simulink model "SRF_DDSRF_Simulink_Imperix"  (R2025a)
settings: Solver=ode45  StartTime=0.0  StopTime=0.3  RelTol=1e-3
PreLoadFcn:
  | % --- DO NOT REMOVE THIS CODE (2024.2.b2) ---
  |     % create Simulink variants
  |     if not(exist('variant_simulation', 'var'))
  |         variant_simulation = Simulink.Variant('SIMULINK_MODE==0');
  |     end
  |     if not(exist('variant_generation', 'var'))
  |         variant_generation = Simulink.Variant('SIMULINK_MODE==1');
  |     end
  | 
  |     % check SDK version
  |     required_lib_version = 3900.3;
  |     required_lib_ver_str = '2024.2.beta2';
  |     lib_path = [getenv('IX_SIMULINK_ACG_BB_3') '\simulink\blocks\BoomBox.slx'];
  |     if exist(lib_path, 'file')
  |         lib_version = str2double(Simulink.MDLInfo(lib_path).ModelVersion); % fullpath to avoid getting shadowing files
  |         if lib_version < required_lib_version || isnan(lib_version)
  |             error(['The model ''' bdroot ''' has been saved with a more recent version of ACG SDK (' required_lib_ver_str ') and might not work as expected. <a href="matlab:private_end_string = ''--- PLACE YOUR CODE BELOW THIS LINE ---'';private_fcn = get_param(bdroot, ''PreLoadFcn'');private_end_index = strfind(private_fcn, private_end_string);set_param(bdroot, ''PreLoadFcn'', strtrim(private_fcn(private_end_index(end)+length(private_end_string):end)));private_fcn = get_param(bdroot, ''PostLoadFcn'');private_end_index = strfind(private_fcn, private_end_string);set_param(bdroot, ''PostLoadFcn'', strtrim(private_fcn(private_end_index(end)+length(private_end_string):end)));private_fcn = get_param(bdroot, ''InitFcn'');private_end_index = strfind(private_fcn, private_end_string);set_param(bdroot, ''InitFcn'', strtrim(private_fcn(private_end_index(end)+length(private_end_string):end)));clear private_end_string private_fcn private_end_index;open(bdroot);">Click here</a> to continue anyway, or download the latest version of the SDK at <a href="www.imperix.com/downloads">www.imperix.ch/downloads</a>.']);
  |         end
  |     elseif exist(getenv('IX_SIMULINK_ACG_BB_3'), 'dir')
  |         error(['Library file for imperix ACG SDK not found in path ''' lib_path '''. Please try to re-install ACG SDK (<a href="www.imperix.com/downloads">www.imperix.ch/downloads</a>).']);
  |     else
  |         error('ACG SDK is not installed on this computer and the model will not work as expected. Please download ACG SDK at <a href="www.imperix.com/downloads">www.imperix.ch/downloads</a>, install it, and reopen the model.');
  |     end
  |     clear required_lib_version required_lib_ver_str lib_path lib_version;
  | 
  |     ix_acg_path = getenv('IX_SIMULINK_ACG_BB_3');
  |     addpath(fullfile(ix_acg_path, 'simulink\target'));
  |     addpath(fullfile(ix_acg_path, 'simulink\blocks'));
  |     addpath(fullfile(ix_acg_path, 'simulink\functions'));
  |     sl_refresh_customizations;
  |     clear ix_acg_path;
  | 
  |     % The SIMULINK_MODE variable is created in the base
  |     % workspace in the PostLoadFcn from the block whose id is kb0101
  |     % All opened models share a common variant configuration.
  | 
  |     Model_PreLoadFcn(bdroot);
  | % --- PLACE YOUR CODE BELOW THIS LINE ---
PostLoadFcn:
  | % --- DO NOT REMOVE THIS CODE (2024.2.b2) ---
  |     % change the execution mode of simulink depending on the radio button:
  |     if(strcmp('Automated Code Generation',get_param(Find_imperix_blocks(bdroot,'Configuration'),'SLMODE')))
  |         assignin('base', 'SIMULINK_MODE', 1);
  |     else
  |         assignin('base', 'SIMULINK_MODE', 0);
  |     end
  | 
  |     Model_PostLoadFcn(bdroot);
  | % --- PLACE YOUR CODE BELOW THIS LINE ---
InitFcn:
  | % --- DO NOT REMOVE THIS CODE (2024.2.b2) ---
  |     % check SDK version
  |     required_lib_version = 3900.3;
  |     required_lib_ver_str = '2024.2.beta2';
  |     lib_path = [getenv('IX_SIMULINK_ACG_BB_3') '\simulink\blocks\BoomBox.slx'];
  |     if exist(lib_path, 'file')
  |         lib_version = str2double(Simulink.MDLInfo(lib_path).ModelVersion); % fullpath to avoid getting shadowing files
  |         if lib_version < required_lib_version || isnan(lib_version)
  |             error(['The model ''' bdroot ''' has been saved with a more recent version of ACG SDK (' required_lib_ver_str ') and might not work as expected. <a href="matlab:private_end_string = ''--- PLACE YOUR CODE BELOW THIS LINE ---'';private_fcn = get_param(bdroot, ''PreLoadFcn'');private_end_index = strfind(private_fcn, private_end_string);set_param(bdroot, ''PreLoadFcn'', strtrim(private_fcn(private_end_index(end)+length(private_end_string):end)));private_fcn = get_param(bdroot, ''PostLoadFcn'');private_end_index = strfind(private_fcn, private_end_string);set_param(bdroot, ''PostLoadFcn'', strtrim(private_fcn(private_end_index(end)+length(private_end_string):end)));private_fcn = get_param(bdroot, ''InitFcn'');private_end_index = strfind(private_fcn, private_end_string);set_param(bdroot, ''InitFcn'', strtrim(private_fcn(private_end_index(end)+length(private_end_string):end)));clear private_end_string private_fcn private_end_index;open(bdroot);">Click here</a> to continue anyway, or download the latest version of the SDK at <a href="www.imperix.com/downloads">www.imperix.ch/downloads</a>.']);
  |         end
  |     elseif exist(getenv('IX_SIMULINK_ACG_BB_3'), 'dir')
  |         error(['Library file for imperix ACG SDK not found in path ''' lib_path '''. Please try to re-install ACG SDK (<a href="www.imperix.com/downloads">www.imperix.ch/downloads</a>).']);
  |     else
  |         error('ACG SDK is not installed on this computer and the model will not work as expected. Please download ACG SDK at <a href="www.imperix.com/downloads">www.imperix.ch/downloads</a>, install it, and reopen the model.');
  |     end
  |     clear required_lib_version required_lib_ver_str lib_path lib_version;
  | 
  |     Model_InitFcn(bdroot);
  | % --- PLACE YOUR CODE BELOW THIS LINE ---
model workspace (MAT data in the model file):
  CTRLPERIOD = [1e-05 5e-06]
  global_cycle_delay = 2e-06
undefined symbols (not defined in the file): DiscIntNeverNeededParam, dspblkCoreblockFVToolHelper, gcbh
libraries: simulink x4, slpidlib x2, BoomBox x2, spsabctodq0Lib x1
settings Model: Creator=matlab  LastModifiedBy=lucaslee
settings SolverCC: AlgebraicLoopSolver=TrustRegion
settings DataIOCC: ReturnWorkspaceOutputs=off
settings OptimizationCC: LifeSpan=inf
settings DebuggingCC: UnconnectedInputMsg=warning  UnconnectedOutputMsg=warning  UnconnectedLineMsg=warning  ArithmeticOperatorsInVariantConditions=warning
settings HardwareCC: ProdBitPerSizeT=32.0  ProdBitPerPtrDiffT=32.0  ProdWordSize=32.0  ProdHWDeviceType=Specified
settings ModelReferenceCC: EnableRefExpFcnMdlSchedulingChecks=on
settings SFSimCC: SimUseLocalCustomCode=off  CustomCodeUndefinedFunction=UseInterfaceOnly
settings RTWCC: RTWUseLocalCustomCode=off  GPUComputeCapability=3.5
settings CodeAppCC: StateflowObjectComments=on
settings SimscapeCC: SimscapeNormalizeSystem=off

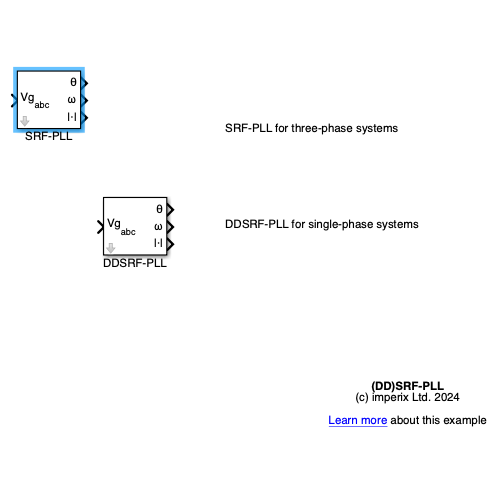
[thumbnail: Simulink's stored preview of the top-level diagram]
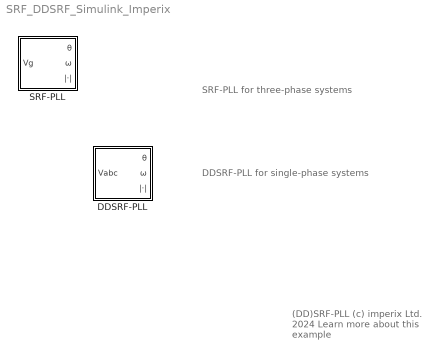
== system SRF_DDSRF_Simulink_Imperix ==
  note: DDSRF-PLL for single-phase systems
  note: SRF-PLL for three-phase systems
  note: (DD)SRF-PLL
      | (c) imperix Ltd. 2024
      |
      | Learn more about this example
  DDSRF-PLL : Subsystem  mask(DSOGI-PLL){FREQ=50, zeta=1/sqrt(2), BW=30, f_LPF=50/sqrt(2), F_out=on, fc=15}
      mask prompts: FREQ "Nominal frequency [Hz]"; zeta "SRF-PLL Damping factor ζ"; BW "SRF-PLL Bandwidth [Hz]"; f_LPF "DDSRF LPF cut off freq. [Hz]"; F_out "Frequency output filter"; fc "LPF cut off frequency [Hz]"
      mask help:
      | This blocks implements a three-phase PLL based on a second order generalized integrator.
      |
      | Return values are in radian [0.2pi[ for the phase, in rad/s for the frequency and in the same unit as the input for the voltage.
      mask Help: https://imperix.com/doc/implementation/synchronous-reference-frame-pll
      mask DialogControl DescGroupVar Prompt: SRF-PLL
      mask DialogControl DescTextVar Prompt: This blocks implements a three phase synchronous reference frame PLL.
      mask DialogControl Control2 Prompt: Return values are in radian [0.2pi[ for the phase, in rad/s for the frequency and in the same unit as the input for the voltage.
      mask DialogControl Container4 Prompt: Parameters
      mask DialogControl Container5 Prompt: Frequency output
      mask Display:
      | %Print the block type:
      | color('black');
      | port_label('input',1,'Vg_{abc}','texmode','on');
      | port_label('output',1,'\theta','texmode','on');
      | port_label('output',2,'\omega','texmode','on');
      | port_label('output',3,'|·|','texmode','on');
  SRF-PLL : Subsystem  mask(DSOGI-PLL){FREQ=50, zeta=1/sqrt(2), BW=30, F_out=on, fc=15}
      mask prompts: FREQ "Nominal frequency [Hz]"; zeta "SRF-PLL Damping factor ζ"; BW "SRF-PLL Bandwidth [Hz]"; F_out "Frequency output filter"; fc "LPF cut off frequency [Hz]"
      mask help:
      | This blocks implements a three-phase PLL based on a second order generalized integrator.
      |
      | Return values are in radian [0.2pi[ for the phase, in rad/s for the frequency and in the same unit as the input for the voltage.
      mask Help: https://imperix.com/doc/implementation/synchronous-reference-frame-pll
      mask DialogControl DescGroupVar Prompt: SRF-PLL
      mask DialogControl DescTextVar Prompt: This blocks implements a three phase synchronous reference frame PLL.
      mask DialogControl Control2 Prompt: Return values are in radian [0.2pi[ for the phase, in rad/s for the frequency and in the same unit as the input for the voltage.
      mask DialogControl Container4 Prompt: Parameters
      mask DialogControl Container5 Prompt: Frequency output
      mask Display:
      | %Print the block type:
      | color('black');
      | port_label('input',1,'Vg_{abc}','texmode','on');
      | port_label('output',1,'\theta','texmode','on');
      | port_label('output',2,'\omega','texmode','on');
      | port_label('output',3,'|·|','texmode','on');

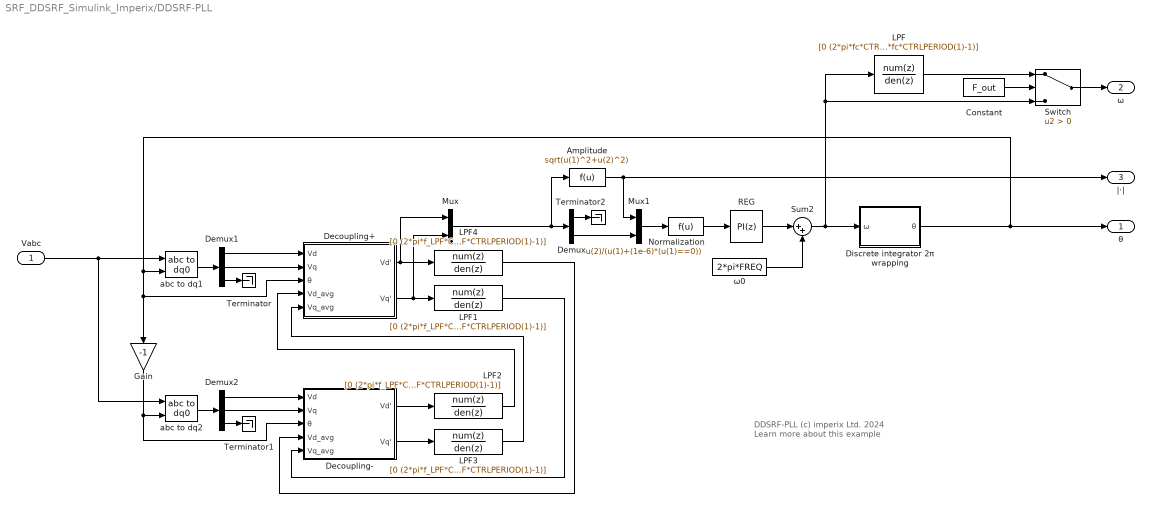
== system SRF_DDSRF_Simulink_Imperix/DDSRF-PLL ==
  note: DDSRF-PLL
      | (c) imperix Ltd. 2024
      |
      | Learn more about this example
  Vabc : Inport
  Amplitude : Fcn  Expr=sqrt(u(1)^2+u(2)^2)
  Constant : Constant  Value=F_out
  Decoupling+ : Subsystem
  Decoupling- : Subsystem
  Demux : Demux  Outputs=2
  Demux1 : Demux  Outputs=3
  Demux2 : Demux  Outputs=3
  Discrete integrator 2π wrapping : Subsystem
  Gain : Gain  Gain=-1
  LPF : DiscreteFilter  Numerator=[0 (2*pi*fc*CTRLPERIOD(1))]  Denominator=[1 (2*pi*fc*CTRLPERIOD(1)-1)]  InitialStates=FREQ/fc/CTRLPERIOD(1)
  LPF1 : DiscreteFilter  Numerator=[0 (2*pi*f_LPF*CTRLPERIOD(1))]  Denominator=[1 (2*pi*f_LPF*CTRLPERIOD(1)-1)]
  LPF2 : DiscreteFilter  Numerator=[0 (2*pi*f_LPF*CTRLPERIOD(1))]  Denominator=[1 (2*pi*f_LPF*CTRLPERIOD(1)-1)]
  LPF3 : DiscreteFilter  Numerator=[0 (2*pi*f_LPF*CTRLPERIOD(1))]  Denominator=[1 (2*pi*f_LPF*CTRLPERIOD(1)-1)]
  LPF4 : DiscreteFilter  Numerator=[0 (2*pi*f_LPF*CTRLPERIOD(1))]  Denominator=[1 (2*pi*f_LPF*CTRLPERIOD(1)-1)]  InitialStates=325/(2*pi*f_LPF)/CTRLPERIOD(1)
  Mux : Mux  Inputs=2
  Mux1 : Mux  Inputs=2
  Normalization : Fcn  Expr=u(2)/(u(1)+(1e-6)*(u(1)==0))
  REG : slpidlib/PID Controller  Controller=PI  Form=Parallel  TimeDomain=Discrete-time  UseExternalTs=off  SampleTime=-1  IntegratorMethod=Trapezoidal  FilterMethod=Forward Euler  ControllerParametersSource=internal  P=2*2*pi*BW*zeta  I=BW*BW*4*pi*pi  UseKiTs=off  D=0  UseExternalDerivativeSource=off  N=100  UseFilter=on  TunerSelectOption=Transfer Function Based (PID Tuner App)  InitialConditionSource=internal  InitialConditionForIntegrator=0  InitialConditionForFilter=0  DifferentiatorICPrevScaledInput=0  ExternalReset=none  TrackingMode=off  Kt=1  LimitOutput=off  SatLimitsSource=internal  UpperSaturationLimit=inf  LowerSaturationLimit=-inf  LinearizeAsGain=on  AntiWindupMode=none  Kb=1  LimitIntegrator=off  UpperIntegratorSaturationLimit=inf  LowerIntegratorSaturationLimit=-inf  POutMin=[]  POutMax=[]  IOutMin=[]  IOutMax=[]  DOutMin=[]  DOutMax=[]  NOutMin=[]  NOutMax=[]  SumOutMin=[]  SumOutMax=[]  SaturationOutMin=[]  SaturationOutMax=[]  PParamMin=[]  PParamMax=[]  IParamMin=[]  IParamMax=[]  DParamMin=[]  DParamMax=[]  NParamMin=[]  NParamMax=[]  KbParamMin=[]  KbParamMax=[]  KtParamMin=[]  KtParamMax=[]  KbOutMin=[]  KbOutMax=[]  KtOutMin=[]  KtOutMax=[]  IntegratorOutMin=[]  IntegratorOutMax=[]  FilterOutMin=[]  FilterOutMax=[]  SumI1OutMin=[]  SumI1OutMax=[]  SumI2OutMin=[]  SumI2OutMax=[]  SumI3OutMin=[]  SumI3OutMax=[]  SumI4OutMin=[]  SumI4OutMax=[]  SumDOutMin=[]  SumDOutMax=[]  DifferentiatorOutMin=[]  DifferentiatorOutMax=[]  FilterDiffOutCoefMin=[]  FilterDiffOutCoefMax=[]  ReciprocalOutMin=[]  ReciprocalOutMax=[]  SumDenOutMin=[]  SumDenOutMax=[]  SumNumOutMin=[]  SumNumOutMax=[]  DivideOutMin=[]  DivideOutMax=[]  UdiffTsProdOutMin=[]  UdiffTsProdOutMax=[]  NTsProdOutMin=[]  NTsProdOutMax=[]  UintegralTsProdOutMin=[]  UintegralTsProdOutMax=[]  UngainTsProdOutMin=[]  UngainTsProdOutMax=[]  ClampingZeroOutDataTypeStr=Inherit: Inherit via back propagation  ClampingZeroOutMin=[]  ClampingZeroOutMax=[]  FilterDenConstantOutDataTypeStr=Inherit: Inherit via back propagation  FilterDenConstantOutMin=[]  FilterDenConstantOutMax=[]  PCopyOutDataTypeStr=Inherit: Inherit via back propagation  PCopyOutMin=[]  PCopyOutMax=[]  NCopyOutDataTypeStr=Inherit: Inherit via back propagation  NCopyOutMin=[]  NCopyOutMax=[]  IntegratorContinuousStateAttributes=''  IntegratorStateMustResolveToSignalObject=off  IntegratorRTWStateStorageClass=Auto  FilterContinuousStateAttributes=''  FilterStateMustResolveToSignalObject=off  FilterRTWStateStorageClass=Auto  ParallelPVariant=InternalParameters  IdealPVariant=Disabled  IVariant=InternalParameters  DVariant=Disabled  IntegratorVariant=Discrete  SatVariant=Disabled  AWVariant=Passthrough  PCopyVariant=Disabled  TRVariant=Disabled  FdbkBlocksVariant=Forward  IdealPFdbkVariant=Disabled  SatFdbkVariant=Disabled  DerivativeFilterVariant=Disabled  NVariant=Disabled  NCopyVariant=Disabled_SignalSpec  FilterICVariant=Disabled  IntegratorICVariant=InternalICs  ExternalResetVariant=Disabled  TRSumVariant=Passthrough  SumFdbkVariant=Disabled  SumVariant=Sum_PI  TsampFilterVariant=InternalTs  TsampNgainVariant=Passthrough  TsampIntegralVariant=Disabled_SignalSpec  ExternalSaturationOutDataTypeStr=Inherit: Same as second input  DerivativeSourceVariant=Disabled  PreIntVariant=InternalPreInt
  Sum2 : Sum  Inputs=|++
  Switch : Switch  Criteria=u2 > Threshold  SaturateOnIntegerOverflow=off  InputSameDT=off
  Terminator : Terminator
  Terminator1 : Terminator
  Terminator2 : Terminator
  abc to dq1 : BoomBox/Transformations/abc to dq0  KBID=kb0601
  abc to dq2 : BoomBox/Transformations/abc to dq0  KBID=kb0601
  ω0 : Constant  Value=2*pi*FREQ  OutDataTypeStr=single
  θ : Outport  OutDataTypeStr=single
  ω : Outport  Port=2  OutDataTypeStr=single
  |·| : Outport  Port=3  OutDataTypeStr=single
  wires:
  ω0/1 -> Sum2/2
  Mux/1 -> Amplitude/1, Demux/1
  Demux/2 -> Mux1/2
  Amplitude/1 -> Mux1/1, |·|/1
  Mux1/1 -> Normalization/1
  Discrete integrator 2π wrapping/1(θ) -> Gain/1, Decoupling+/3(θ), abc to dq1/2, θ/1
  Normalization/1 -> REG/1
  REG/1 -> Sum2/1
  Switch/1 -> ω/1
  Constant/1 -> Switch/2
  Sum2/1 -> Discrete integrator 2π wrapping/1(ω), LPF/1, Switch/3
  abc to dq1/1 -> Demux1/1
  Demux1/1 -> Decoupling+/1(Vd)
  Demux1/2 -> Decoupling+/2(Vq)
  abc to dq2/1 -> Demux2/1
  Demux2/1 -> Decoupling-/1(Vd)
  Demux2/2 -> Decoupling-/2(Vq)
  Vabc/1 -> abc to dq1/1, abc to dq2/1
  Decoupling-/1(Vd') -> LPF2/1
  Decoupling-/2(Vq') -> LPF3/1
  Decoupling+/1(Vd') -> Mux/1, LPF4/1
  Decoupling+/2(Vq') -> Mux/2, LPF1/1
  LPF1/1 -> Decoupling-/5(Vq_avg)
  LPF4/1 -> Decoupling-/4(Vd_avg)
  Gain/1 -> Decoupling-/3(θ), abc to dq2/2
  Demux1/3 -> Terminator/1
  Demux2/3 -> Terminator1/1
  LPF/1 -> Switch/1
  Demux/1 -> Terminator2/1
  LPF2/1 -> Decoupling+/4(Vd_avg)
  LPF3/1 -> Decoupling+/5(Vq_avg)

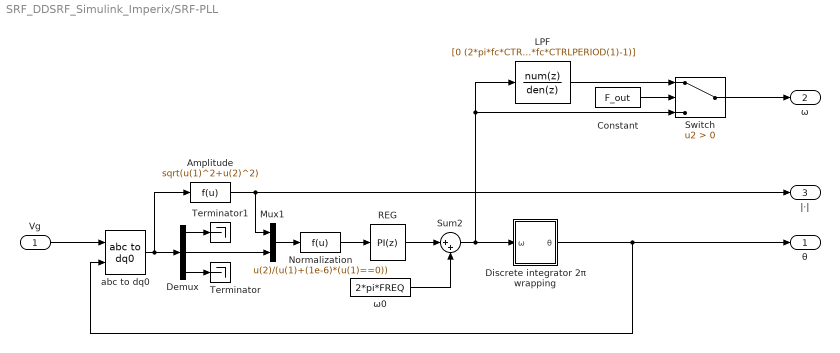
== system SRF_DDSRF_Simulink_Imperix/SRF-PLL ==
  Vg : Inport
  Amplitude : Fcn  Expr=sqrt(u(1)^2+u(2)^2)
  Constant : Constant  Value=F_out
  Demux : Demux  Outputs=3
  Discrete integrator 2π wrapping : Subsystem
  LPF : DiscreteFilter  LoadFcn=dspblkCoreblockFVToolHelper(gcbh,'load');  Numerator=[0 (2*pi*fc*CTRLPERIOD(1))]  Denominator=[1 (2*pi*fc*CTRLPERIOD(1)-1)]  InitialStates=FREQ/fc/CTRLPERIOD(1)
      settings: CopyFcn=dspblkCoreblockFVToolHelper(gcbh,'copy');  DeleteFcn=dspblkCoreblockFVToolHelper(gcbh,'close');  ModelCloseFcn=dspblkCoreblockFVToolHelper(gcbh,'close');  PreSaveFcn=dspblkCoreblockFVToolHelper(gcbh,'presave');  PostSaveFcn=dspblkCoreblockFVToolHelper(gcbh,'postsave');  CloseFcn=dspblkCoreblockFVToolHelper(gcbh,'close');
  Mux1 : Mux  Inputs=2
  Normalization : Fcn  Expr=u(2)/(u(1)+(1e-6)*(u(1)==0))
  REG : slpidlib/PID Controller  Controller=PI  Form=Parallel  TimeDomain=Discrete-time  UseExternalTs=off  SampleTime=-1  IntegratorMethod=Trapezoidal  FilterMethod=Forward Euler  ControllerParametersSource=internal  P=2*2*pi*BW*zeta  I=BW*BW*4*pi*pi  UseKiTs=off  D=0  UseExternalDerivativeSource=off  N=100  UseFilter=on  TunerSelectOption=Transfer Function Based (PID Tuner App)  InitialConditionSource=internal  InitialConditionForIntegrator=0  InitialConditionForFilter=0  DifferentiatorICPrevScaledInput=0  ExternalReset=none  TrackingMode=off  Kt=1  LimitOutput=off  SatLimitsSource=internal  UpperSaturationLimit=inf  LowerSaturationLimit=-inf  LinearizeAsGain=on  AntiWindupMode=none  Kb=1  LimitIntegrator=off  UpperIntegratorSaturationLimit=inf  LowerIntegratorSaturationLimit=-inf  POutMin=[]  POutMax=[]  IOutMin=[]  IOutMax=[]  DOutMin=[]  DOutMax=[]  NOutMin=[]  NOutMax=[]  SumOutMin=[]  SumOutMax=[]  SaturationOutMin=[]  SaturationOutMax=[]  PParamMin=[]  PParamMax=[]  IParamMin=[]  IParamMax=[]  DParamMin=[]  DParamMax=[]  NParamMin=[]  NParamMax=[]  KbParamMin=[]  KbParamMax=[]  KtParamMin=[]  KtParamMax=[]  KbOutMin=[]  KbOutMax=[]  KtOutMin=[]  KtOutMax=[]  IntegratorOutMin=[]  IntegratorOutMax=[]  FilterOutMin=[]  FilterOutMax=[]  SumI1OutMin=[]  SumI1OutMax=[]  SumI2OutMin=[]  SumI2OutMax=[]  SumI3OutMin=[]  SumI3OutMax=[]  SumI4OutMin=[]  SumI4OutMax=[]  SumDOutMin=[]  SumDOutMax=[]  DifferentiatorOutMin=[]  DifferentiatorOutMax=[]  FilterDiffOutCoefMin=[]  FilterDiffOutCoefMax=[]  ReciprocalOutMin=[]  ReciprocalOutMax=[]  SumDenOutMin=[]  SumDenOutMax=[]  SumNumOutMin=[]  SumNumOutMax=[]  DivideOutMin=[]  DivideOutMax=[]  UdiffTsProdOutMin=[]  UdiffTsProdOutMax=[]  NTsProdOutMin=[]  NTsProdOutMax=[]  UintegralTsProdOutMin=[]  UintegralTsProdOutMax=[]  UngainTsProdOutMin=[]  UngainTsProdOutMax=[]  ClampingZeroOutDataTypeStr=Inherit: Inherit via back propagation  ClampingZeroOutMin=[]  ClampingZeroOutMax=[]  FilterDenConstantOutDataTypeStr=Inherit: Inherit via back propagation  FilterDenConstantOutMin=[]  FilterDenConstantOutMax=[]  PCopyOutDataTypeStr=Inherit: Inherit via back propagation  PCopyOutMin=[]  PCopyOutMax=[]  NCopyOutDataTypeStr=Inherit: Inherit via back propagation  NCopyOutMin=[]  NCopyOutMax=[]  IntegratorContinuousStateAttributes=''  IntegratorStateMustResolveToSignalObject=off  IntegratorRTWStateStorageClass=Auto  FilterContinuousStateAttributes=''  FilterStateMustResolveToSignalObject=off  FilterRTWStateStorageClass=Auto  ParallelPVariant=InternalParameters  IdealPVariant=Disabled  IVariant=InternalParameters  DVariant=Disabled  IntegratorVariant=Discrete  SatVariant=Disabled  AWVariant=Passthrough  PCopyVariant=Disabled  TRVariant=Disabled  FdbkBlocksVariant=Forward  IdealPFdbkVariant=Disabled  SatFdbkVariant=Disabled  DerivativeFilterVariant=Disabled  NVariant=Disabled  NCopyVariant=Disabled_SignalSpec  FilterICVariant=Disabled  IntegratorICVariant=InternalICs  ExternalResetVariant=Disabled  TRSumVariant=Passthrough  SumFdbkVariant=Disabled  SumVariant=Sum_PI  TsampFilterVariant=InternalTs  TsampNgainVariant=Passthrough  TsampIntegralVariant=Disabled_SignalSpec  ExternalSaturationOutDataTypeStr=Inherit: Same as second input  DerivativeSourceVariant=Disabled  PreIntVariant=InternalPreInt
  Sum2 : Sum  Inputs=|++
  Switch : Switch  Criteria=u2 > Threshold  SaturateOnIntegerOverflow=off  InputSameDT=off
  Terminator : Terminator
  Terminator1 : Terminator
  abc to dq0 : spsabctodq0Lib/abc to dq0  Alignment=90 degrees behind phase A axis
  ω0 : Constant  Value=2*pi*FREQ  OutDataTypeStr=single
  θ : Outport  OutDataTypeStr=single
  ω : Outport  Port=2  OutDataTypeStr=single
  |·| : Outport  Port=3  OutDataTypeStr=single
  wires:
  ω0/1 -> Sum2/2
  abc to dq0/1 -> Demux/1, Amplitude/1
  Amplitude/1 -> Mux1/1, |·|/1
  Mux1/1 -> Normalization/1
  Discrete integrator 2π wrapping/1(θ) -> abc to dq0/2, θ/1
  Normalization/1 -> REG/1
  REG/1 -> Sum2/1
  Vg/1 -> abc to dq0/1
  Sum2/1 -> Discrete integrator 2π wrapping/1(ω), LPF/1, Switch/3
  LPF/1 -> Switch/1
  Switch/1 -> ω/1
  Constant/1 -> Switch/2
  Demux/3 -> Terminator/1
  Demux/1 -> Terminator1/1
  Demux/2 -> Mux1/2

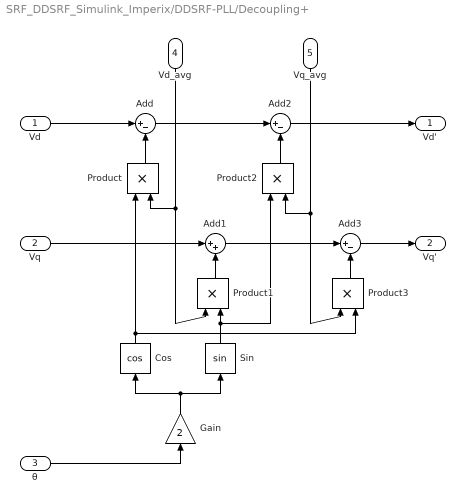
== system SRF_DDSRF_Simulink_Imperix/DDSRF-PLL/Decoupling+ ==
  Vd : Inport
  Vq : Inport  Port=2
  θ : Inport  Port=3
  Vd_avg : Inport  Port=4
  Vq_avg : Inport  Port=5
  Add : Sum  Inputs=|+-
  Add1 : Sum  Inputs=|++
  Add2 : Sum  Inputs=|+-
  Add3 : Sum  Inputs=|+-
  Cos : Trigonometry  Operator=cos
  Gain : Gain  Gain=2
  Product{,1..3} (4 alike) : Product
  Sin : Trigonometry
  Vd' : Outport
  Vq' : Outport  Port=2
  wires:
  θ/1 -> Gain/1
  Gain/1 -> Sin/1, Cos/1
  Cos/1 -> Product3/2, Product/1
  Product/1 -> Add/2
  Vd/1 -> Add/1
  Sin/1 -> Product2/1, Product1/2
  Vd_avg/1 -> Product/2, Product1/1
  Product1/1 -> Add1/2
  Vq/1 -> Add1/1
  Vq_avg/1 -> Product2/2, Product3/1
  Product2/1 -> Add2/2
  Add/1 -> Add2/1
  Add2/1 -> Vd'/1
  Product3/1 -> Add3/2
  Add1/1 -> Add3/1
  Add3/1 -> Vq'/1

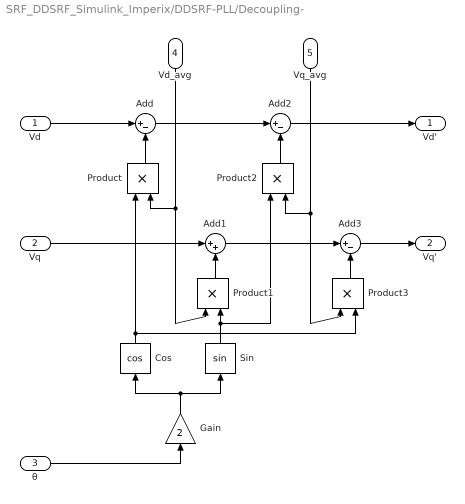
== system SRF_DDSRF_Simulink_Imperix/DDSRF-PLL/Decoupling- ==
  Vd : Inport
  Vq : Inport  Port=2
  θ : Inport  Port=3
  Vd_avg : Inport  Port=4
  Vq_avg : Inport  Port=5
  Add : Sum  Inputs=|+-
  Add1 : Sum  Inputs=|++
  Add2 : Sum  Inputs=|+-
  Add3 : Sum  Inputs=|+-
  Cos : Trigonometry  Operator=cos
  Gain : Gain  Gain=2
  Product{,1..3} (4 alike) : Product
  Sin : Trigonometry
  Vd' : Outport
  Vq' : Outport  Port=2
  wires:
  θ/1 -> Gain/1
  Gain/1 -> Sin/1, Cos/1
  Cos/1 -> Product3/2, Product/1
  Product/1 -> Add/2
  Vd/1 -> Add/1
  Sin/1 -> Product2/1, Product1/2
  Vd_avg/1 -> Product/2, Product1/1
  Product1/1 -> Add1/2
  Vq/1 -> Add1/1
  Vq_avg/1 -> Product2/2, Product3/1
  Product2/1 -> Add2/2
  Add/1 -> Add2/1
  Add2/1 -> Vd'/1
  Product3/1 -> Add3/2
  Add1/1 -> Add3/1
  Add3/1 -> Vq'/1

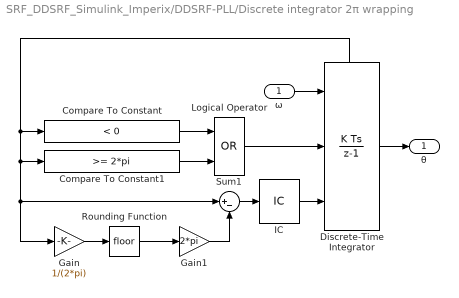
== system SRF_DDSRF_Simulink_Imperix/DDSRF-PLL/Discrete integrator 2π wrapping ==
  ω : Inport
  Compare To Constant : simulink/Logic and Bit Operations/Compare To Constant  relop=<  const=0  OutDataTypeStr=boolean
  Compare To Constant1 : simulink/Logic and Bit Operations/Compare To Constant  relop=>=  const=2*pi  OutDataTypeStr=boolean
  Discrete-Time Integrator : DiscreteIntegrator  ExternalReset=sampled level  InitialConditionSource=external  SampleTime=-1  ShowStatePort=on  ICPrevOutput=DiscIntNeverNeededParam  ICPrevScaledInput=DiscIntNeverNeededParam
  Gain : Gain  Gain=1/(2*pi)
      settings: AttributesFormatString=%<Gain>
  Gain1 : Gain  Gain=2*pi
  IC : InitialCondition  Value=0
  Logical Operator : Logic  Operator=OR  AllPortsSameDT=off  OutDataTypeStr=boolean
  Rounding Function : Rounding
  Sum1 : Sum  Inputs=|+-
  θ : Outport
  wires:
  Gain1/1 -> Sum1/2
  Gain/1 -> Rounding Function/1
  IC/1 -> Discrete-Time Integrator/3
  Compare To Constant1/1 -> Logical Operator/2
  Discrete-Time Integrator/State -> Compare To Constant1/1, Sum1/1, Gain/1, Compare To Constant/1
  Compare To Constant/1 -> Logical Operator/1
  Logical Operator/1 -> Discrete-Time Integrator/2
  Sum1/1 -> IC/1
  Rounding Function/1 -> Gain1/1
  ω/1 -> Discrete-Time Integrator/1
  Discrete-Time Integrator/1 -> θ/1

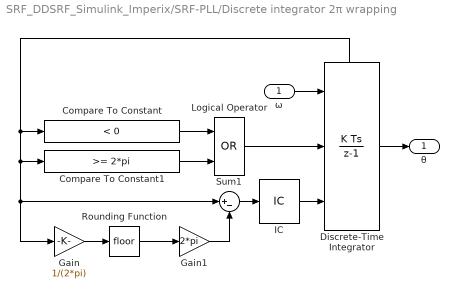
== system SRF_DDSRF_Simulink_Imperix/SRF-PLL/Discrete integrator 2π wrapping ==
  ω : Inport
  Compare To Constant : simulink/Logic and Bit Operations/Compare To Constant  relop=<  const=0  OutDataTypeStr=boolean
  Compare To Constant1 : simulink/Logic and Bit Operations/Compare To Constant  relop=>=  const=2*pi  OutDataTypeStr=boolean
  Discrete-Time Integrator : DiscreteIntegrator  ExternalReset=sampled level  InitialConditionSource=external  SampleTime=-1  ShowStatePort=on  ICPrevOutput=DiscIntNeverNeededParam  ICPrevScaledInput=DiscIntNeverNeededParam
  Gain : Gain  Gain=1/(2*pi)
      settings: AttributesFormatString=%<Gain>
  Gain1 : Gain  Gain=2*pi
  IC : InitialCondition  Value=0
  Logical Operator : Logic  Operator=OR  AllPortsSameDT=off  OutDataTypeStr=boolean
  Rounding Function : Rounding
  Sum1 : Sum  Inputs=|+-
  θ : Outport
  wires:
  Gain1/1 -> Sum1/2
  Gain/1 -> Rounding Function/1
  IC/1 -> Discrete-Time Integrator/3
  Compare To Constant1/1 -> Logical Operator/2
  Discrete-Time Integrator/State -> Compare To Constant1/1, Sum1/1, Gain/1, Compare To Constant/1
  Compare To Constant/1 -> Logical Operator/1
  Logical Operator/1 -> Discrete-Time Integrator/2
  Sum1/1 -> IC/1
  Rounding Function/1 -> Gain1/1
  ω/1 -> Discrete-Time Integrator/1
  Discrete-Time Integrator/1 -> θ/1
